simulink model "LEGO_DC_Motor"  (R2013b)
settings: Solver=ode3  SolverMode=SingleTasking  StartTime=0.0  StopTime=50  FixedStep=ts1  RelTol=1e-3
PostLoadFcn:
  | Ts = 0.1;
  | ts1 = 0.004;
  | a_d = 0.8;
InitFcn:
  | Ts = 0.1;
  | ts1 = 0.004;
  | a_d = 0.8;
undefined symbols (not defined in the file): kp, sigbuilder_block
libraries: legonxtlib x6, simulink x1, slident x1
CloseFcn:
  | clear Ts ts1 a_d
settings Model: SimulationMode=external  ExtModeTrigDuration=2  Creator=Alphonso Monk  LastModifiedBy=Alphonso Monk
settings OptimizationCC: OptimizeModelRefInitCode=on  LifeSpan=1
settings DebuggingCC: SolverPrmCheckMsg=none
settings HardwareCC: ProdLargestAtomicInteger=Long  ProdLargestAtomicFloat=Float  ProdEndianess=LittleEndian  ProdHWDeviceType=ARM Compatible->ARM 7
settings RTWCC: SystemTargetFile=realtime.tlc  GenerateMakefile=off  TemplateMakefile=realtime.tmf  Description=Run on Target Hardware  RTWVerbose=off  ProcessScript=realtime_make_rtw_hook
settings STFCustomTargetCC: TargetLibSuffix=.a  GenerateSampleERTMain=on  ERTCustomFileBanners=on  SupportNonInlinedSFcns=off  SupportVariableSizeSignals=on  MATLABClassNameForMDSCustomization=Simulink.SoftwareTarget.ERTCustomization  GRTInterface=off  SystemTargetFile=realtime.tlc
settings ERTTargetCC: CodeReplacementLibrary=ANSI_C  GenerateSampleERTMain=on  ParMdlRefBuildCompliant=off  CompOptLevelCompliant=off  ConcurrentExecutionCompliant=off  CombineOutputUpdateFcns=off  ERTFirstTimeCompliant=off  SupportContinuousTime=on  SupportVariableSizeSignals=on  ModelStepFunctionPrototypeControlCompliant=off  CPPClassGenCompliant=off  ExtMode=on  ExtModeTransport=2  ExtModeMexArgs=0 3 9600 30  InlinedParameterPlacement=NonHierarchical  ERTSrcFileBannerTemplate=realtime_code_template.cgt  ERTHdrFileBannerTemplate=realtime_code_template.cgt  ERTDataSrcFileTemplate=realtime_code_template.cgt  ERTDataHdrFileTemplate=realtime_code_template.cgt  ERTCustomFileTemplate=realtime_file_process.tlc

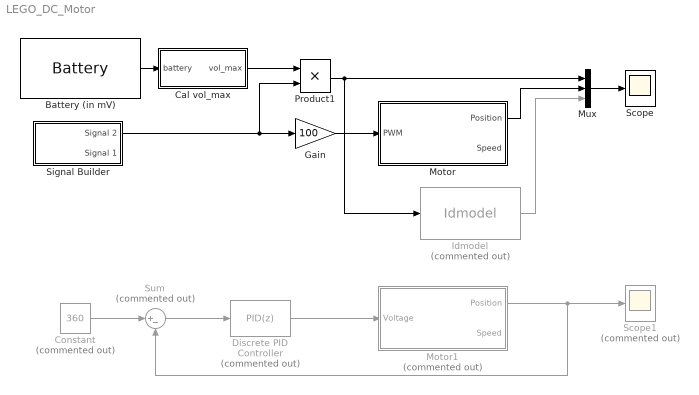
== system LEGO_DC_Motor ==
  Battery (in mV) : legonxtlib/Battery  sampleTime=Ts
  Cal vol_max : Subsystem
  Constant : Constant  Commented=on  Value=360
  Discrete PID Controller : simulink/Continuous/PID Controller  Commented=on  Controller=PID  TimeDomain=Discrete-time  SampleTime=ts1  IntegratorMethod=Forward Euler  FilterMethod=Forward Euler  Form=Parallel  P=kp  I=0  D=0  N=100  InitialConditionSource=internal  InitialConditionForIntegrator=0  InitialConditionForFilter=0  ExternalReset=none  LimitOutput=on  UpperSaturationLimit=9  LowerSaturationLimit=-9  LinearizeAsGain=off  AntiWindupMode=none  Kb=1  TrackingMode=off  Kt=1  PParamMin=[]  PParamMax=[]  IParamMin=[]  IParamMax=[]  DParamMin=[]  DParamMax=[]  NParamMin=[]  NParamMax=[]  KbParamMin=[]  KbParamMax=[]  KtParamMin=[]  KtParamMax=[]  POutMin=[]  POutMax=[]  IOutMin=[]  IOutMax=[]  DOutMin=[]  DOutMax=[]  NOutMin=[]  NOutMax=[]  KbOutMin=[]  KbOutMax=[]  KtOutMin=[]  KtOutMax=[]  IntegratorOutMin=[]  IntegratorOutMax=[]  FilterOutMin=[]  FilterOutMax=[]  SumOutMin=[]  SumOutMax=[]  SumI1OutMin=[]  SumI1OutMax=[]  SumI2OutMin=[]  SumI2OutMax=[]  SumI3OutMin=[]  SumI3OutMax=[]  SumDOutMin=[]  SumDOutMax=[]  SaturationOutMin=[]  SaturationOutMax=[]  IntegratorContinuousStateAttributes=''  IntegratorStateMustResolveToSignalObject=off  IntegratorRTWStateStorageClass=Auto  FilterContinuousStateAttributes=''  FilterStateMustResolveToSignalObject=off  FilterRTWStateStorageClass=Auto
  Gain : Gain  Gain=100
  "Idmodel " : slident/Idmodel   Commented=on  sys=tf1  IC=0  noi=off  seed=[]
  Motor : Subsystem
  Motor1 : Subsystem  Commented=on
  Mux : Mux  Inputs=3
  Product1 : Product  Inputs=**
  Scope : Scope
      settings: SaveName=motorResponse
  Scope1 : Scope  Commented=on
      settings: YMin=353  YMax=353  SaveName=motorResponse1
  Signal Builder : Subsystem  Tag=STV Subsys  LoadFcn=sigbuilder_block('load');  StartFcn=sigbuilder_block('start');  StopFcn=sigbuilder_block('stop');  ClipboardFcn=sigbuilder_block('clipboard');  mask(Sigbuilder block){}
      mask help: Simulink:masks:SigbuilderBlock_MD
      mask init:
      | if ~strcmp(get_param(bdroot(gcbh),'SimulationStatus'),'stopped') tuvar = sigbuilder_block('maskInit'); end
      settings: CopyFcn=sigbuilder_block('copy');  DeleteFcn=sigbuilder_block('delete');  ModelCloseFcn=sigbuilder_block('modelClose');  PreSaveFcn=sigbuilder_block('preSave');  PauseFcn=sigbuilder_block('pause');  ContinueFcn=sigbuilder_block('continue');  NameChangeFcn=sigbuilder_block('namechange');  OpenFcn=sigbuilder_block('open',[6 28.5 1008 484.5 ]);  CloseFcn=sigbuilder_block('close');
      mask Display: plot(0, 0, 100, 100,[2, 2, 32, 32, 2], [68, 8, 8, 68, 68],[32, 2], [38, 38], [32, 19, 2],[53, 60, 44], [32, 17, 17, 2],[16, 16, 31, 31]);txt = getActiveGroup(gcbh);text(2, 100, txt,'verticalAlignment', 'top');
  Sum : Sum  Commented=on  Inputs=|+-
  wires:
  Mux/1 -> Scope/1
  Motor/1(Position) -> Mux/2
  Signal Builder/1(Signal 2) -> Gain/1, Product1/2
  Gain/1 -> Motor/1(PWM)
  Cal vol_max/1(vol_max) -> Product1/1
  Battery (in mV)/1 -> Cal vol_max/1(battery)
  Constant/1 -> Sum/1
  Discrete PID Controller/1 -> Motor1/1(Voltage)
  "Idmodel "/1 -> Mux/3
  Product1/1 -> "Idmodel "/1, Mux/1
  Motor1/1(Position) -> Sum/2, Scope1/1
  Sum/1 -> Discrete PID Controller/1

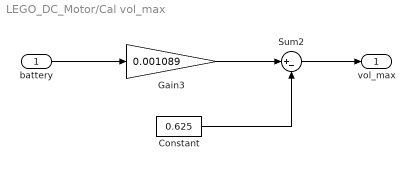
== system LEGO_DC_Motor/Cal vol_max ==
  battery : Inport
  Constant : Constant  Value=0.625  OutDataTypeStr=single
      settings: AttributesFormatString=DataType = %<OutDataTypeStr>
  Gain3 : Gain  Gain=0.001089  OutDataTypeStr=Inherit: Same as input  ParamDataTypeStr=Inherit: Same as input
  Sum2 : Sum  Inputs=|+-  OutDataTypeStr=Inherit: Same as first input
  vol_max : Outport
  wires:
  Gain3/1 -> Sum2/1
  Sum2/1 -> vol_max/1
  Constant/1 -> Sum2/2
  battery/1 -> Gain3/1

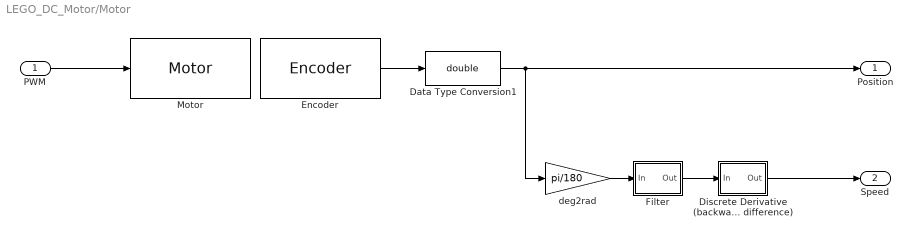
== system LEGO_DC_Motor/Motor ==
  PWM : Inport
  Data Type Conversion1 : DataTypeConversion  OutDataTypeStr=double
  Discrete Derivative (backward difference) : Subsystem
  Encoder : legonxtlib/Encoder  portNumber=B  opMode=No reset  sampleTime=ts1
  Filter : Subsystem
  Motor : legonxtlib/Motor  sportNumber=B  sstopAction=Brake
  deg2rad : Gain  Gain=pi/180  OutDataTypeStr=Inherit: Same as input  ParamDataTypeStr=Inherit: Same as input
  Position : Outport
  Speed : Outport  Port=2
  wires:
  Discrete Derivative (backward difference)/1(Out) -> Speed/1
  PWM/1 -> Motor/1
  Filter/1(Out) -> Discrete Derivative (backward difference)/1(In)
  deg2rad/1 -> Filter/1(In)
  Data Type Conversion1/1 -> Position/1, deg2rad/1
  Encoder/1 -> Data Type Conversion1/1

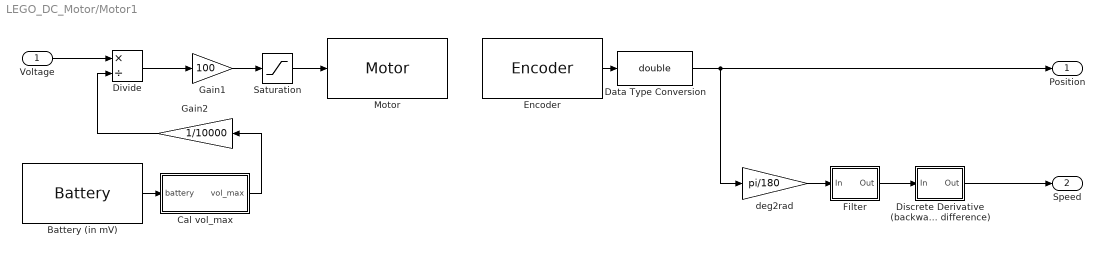
== system LEGO_DC_Motor/Motor1 ==
  Voltage : Inport
  Battery (in mV) : legonxtlib/Battery  sampleTime=Ts
  Cal vol_max : Subsystem
  Data Type Conversion : DataTypeConversion  OutDataTypeStr=double
  Discrete Derivative (backward difference) : Subsystem
  Divide : Product  Inputs=*/
  Encoder : legonxtlib/Encoder  portNumber=B  opMode=No reset  sampleTime=ts1
  Filter : Subsystem
  Gain1 : Gain  Gain=100
  Gain2 : Gain  Gain=1/10000
  Motor : legonxtlib/Motor  sportNumber=B  sstopAction=Brake
  Saturation : Saturate  UpperLimit=100  LowerLimit=-100
  deg2rad : Gain  Gain=pi/180  OutDataTypeStr=Inherit: Same as input  ParamDataTypeStr=Inherit: Same as input
  Position : Outport
  Speed : Outport  Port=2
  wires:
  Encoder/1 -> Data Type Conversion/1
  Data Type Conversion/1 -> Position/1, deg2rad/1
  deg2rad/1 -> Filter/1(In)
  Filter/1(Out) -> Discrete Derivative (backward difference)/1(In)
  Discrete Derivative (backward difference)/1(Out) -> Speed/1
  Cal vol_max/1(vol_max) -> Gain2/1
  Battery (in mV)/1 -> Cal vol_max/1(battery)
  Voltage/1 -> Divide/1
  Saturation/1 -> Motor/1
  Divide/1 -> Gain1/1
  Gain2/1 -> Divide/2
  Gain1/1 -> Saturation/1

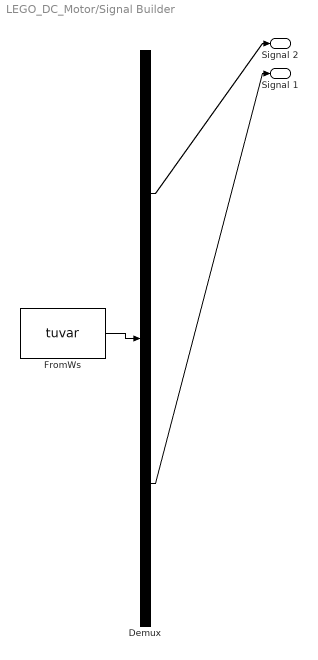
== system LEGO_DC_Motor/Signal Builder ==
  Demux : Demux  Tag=STV Demux  Outputs=2
  FromWs : FromWorkspace  Tag=STV FromWs  VariableName=tuvar  SampleTime=0
      SigBuilderData=|
      | common.afterFinalStr = 'Extrapolate'
      | common.sampleTime = 0
      | dataSet.timeRange = [0 50]
      | dataSet.name = 'SysIdent'
      | sbobj.Groups.Name = 'SysIdent'
      | sbobj.Groups.Signals(1).Name = 'Signal 2'
      | sbobj.Groups.Signals(1).XData = [0 0.5 0.5 1 1 1.5 1.5 2 2 2.5 2.5 3 3 4.5 4.5 6 6 6.5 6.5 7 7 8.5 8.5 10 10 10.5 10.5 11 11 12.5 12.5 14 14 14.5 14.5 15 15 15.5 15.5 17.5 17.5 19 19 19.5 19.5 20.5 20.5 21 21 21.5 21.5 25.5 25.5 26.5 26.5 28 28 28.5 28.5 29.5 29.5 30 30 32.5 32.5 34 34 35.5 35.5 36 36 37.5 37.5 39 39 39.5 39.5 40 40 40.5 40.5 41 41 41.5 41.5 42 42 43 43 44 44 44.5 44.5 45.5 45.5 47.5 47.5 50]
      | sbobj.Groups.Signals(1).YData = [1 1 -1 -1 1 1 -1 -1 1 1 -1 -1 1 1 -1 -1 1 1 -1 -1 1 1 -1 -1 1 1 -1 -1 1 1 -1 -1 1 1 -1 -1 1 1 -1 -1 1 1 -1 -1 1 1 -1 -1 1 1 -1 -1 1 1 -1 -1 1 1 -1 -1 1 1 -1 -1 1 1 -1 -1 1 1 -1 -1 1 1 -1 -1 1 1 -1 -1 1 1 -1 -1 1 1 -1 -1 1 1 -1 -1 1 1 -1 -1 1 1]
      | sbobj.Groups.Signals(2).Name = 'Signal 1'
      | sbobj.Groups.Signals(2).XData = [0 4.95 4.95 9.45 9.45 50]
      | sbobj.Groups.Signals(2).YData = [0 0 1 1 0 0]
      | sbobj.Groups.TimeRange = [0 50]
  Signal 2 : Outport  Tag=STV Outport
  Signal 1 : Outport  Tag=STV Outport  Port=2
  wires:
  FromWs/1 -> Demux/1
  Demux/1 -> Signal 2/1
  Demux/2 -> Signal 1/1

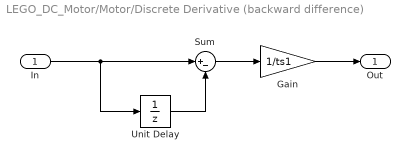
== system LEGO_DC_Motor/Motor/Discrete Derivative (backward difference) ==
  In : Inport
  Gain : Gain  Gain=1/ts1  OutDataTypeStr=Inherit: Same as input  ParamDataTypeStr=Inherit: Same as input
  Sum : Sum  Inputs=|+-  OutDataTypeStr=Inherit: Same as first input
  Unit Delay : UnitDelay  SampleTime=-1
  Out : Outport
  wires:
  Gain/1 -> Out/1
  In/1 -> Sum/1, Unit Delay/1
  Unit Delay/1 -> Sum/2
  Sum/1 -> Gain/1

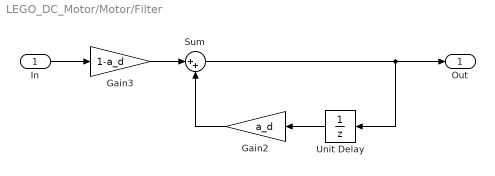
== system LEGO_DC_Motor/Motor/Filter ==
  In : Inport
  Gain2 : Gain  Gain=a_d  OutDataTypeStr=Inherit: Same as input  ParamDataTypeStr=Inherit: Same as input
  Gain3 : Gain  Gain=1-a_d  OutDataTypeStr=Inherit: Same as input  ParamDataTypeStr=Inherit: Same as input
  Sum : Sum  Inputs=|++  OutDataTypeStr=Inherit: Same as first input
  Unit Delay : UnitDelay  SampleTime=-1
  Out : Outport
  wires:
  In/1 -> Gain3/1
  Gain3/1 -> Sum/1
  Gain2/1 -> Sum/2
  Unit Delay/1 -> Gain2/1
  Sum/1 -> Out/1, Unit Delay/1

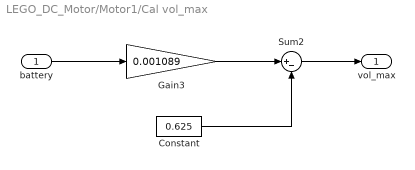
== system LEGO_DC_Motor/Motor1/Cal vol_max ==
  battery : Inport
  Constant : Constant  Value=0.625  OutDataTypeStr=single
      settings: AttributesFormatString=DataType = %<OutDataTypeStr>
  Gain3 : Gain  Gain=0.001089  OutDataTypeStr=Inherit: Same as input  ParamDataTypeStr=Inherit: Same as input
  Sum2 : Sum  Inputs=|+-  OutDataTypeStr=Inherit: Same as first input
  vol_max : Outport
  wires:
  Gain3/1 -> Sum2/1
  Sum2/1 -> vol_max/1
  Constant/1 -> Sum2/2
  battery/1 -> Gain3/1

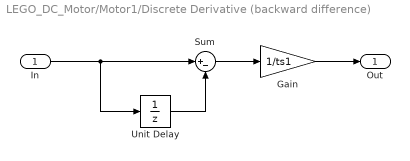
== system LEGO_DC_Motor/Motor1/Discrete Derivative (backward difference) ==
  In : Inport
  Gain : Gain  Gain=1/ts1  OutDataTypeStr=Inherit: Same as input  ParamDataTypeStr=Inherit: Same as input
  Sum : Sum  Inputs=|+-  OutDataTypeStr=Inherit: Same as first input
  Unit Delay : UnitDelay  SampleTime=-1
  Out : Outport
  wires:
  Sum/1 -> Gain/1
  Unit Delay/1 -> Sum/2
  In/1 -> Unit Delay/1, Sum/1
  Gain/1 -> Out/1

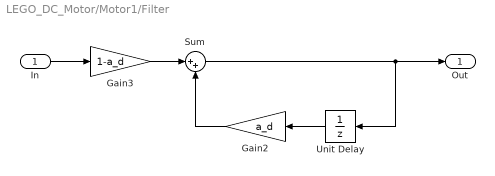
== system LEGO_DC_Motor/Motor1/Filter ==
  In : Inport
  Gain2 : Gain  Gain=a_d  OutDataTypeStr=Inherit: Same as input  ParamDataTypeStr=Inherit: Same as input
  Gain3 : Gain  Gain=1-a_d  OutDataTypeStr=Inherit: Same as input  ParamDataTypeStr=Inherit: Same as input
  Sum : Sum  Inputs=|++  OutDataTypeStr=Inherit: Same as first input
  Unit Delay : UnitDelay  SampleTime=-1
  Out : Outport
  wires:
  Sum/1 -> Unit Delay/1, Out/1
  Unit Delay/1 -> Gain2/1
  Gain2/1 -> Sum/2
  Gain3/1 -> Sum/1
  In/1 -> Gain3/1
